simulink model "Robot2_SDT"  (R2025b)
settings: Solver=VariableStepAuto  StartTime=0.0  StopTime=10.0  RelTol=1e-3
values from neighbouring files (symbols this model uses):
  CoM_variation_x = ureal('CoMx',0,"PlusMinus",[-10e-3 10e-3])    [Satellite_Data.m]
  CoM_variation_y = ureal('CoMy',0,"PlusMinus",[-10e-3 10e-3])    [Satellite_Data.m]
  CoM_variation_z = ureal('CoMz',0,"PlusMinus",[-20e-3 20e-3])    [Satellite_Data.m]
  Cross_section_beam = width_beam*height_beam    (= 0.04)    [Satellite_Data.m]
  Iy_beam = (height_beam*width_beam.^3)/12    [Satellite_Data.m]
  Iz_beam = (width_beam*height_beam.^3)/12    [Satellite_Data.m]
  J_B_B = [J_B_Bxx J_B_Bxy J_B_Bxz;         J_B_Bxy J_B_Byy J_B_Byz;         J_B_Bxz J_B_Byz J_B_Bzz]    [Satellite_Data.m]
  J_C_C = [J_C_Cxx J_C_Cxy J_C_Cxz;         J_C_Cxy J_C_Cyy J_C_Cyz;         J_C_Cxz J_C_Cyz J_C_Czz]    [Satellite_Data.m]
  J_P_P = [J_P_Pxx J_P_Pxy J_P_Pxz;         J_P_Pxy J_P_Pyy J_P_Pyz;         J_P_Pxz J_P_Pyz J_P_Pzz]    [Satellite_Data.m]
  length_beam = 4.7    [Satellite_Data.m]
  m_B = ureal('m_B',1000,'percent',10)    [Satellite_Data.m]
  m_C = ureal('m_C',500,'percent',10)    [Satellite_Data.m]
  m_P = ureal('m_P',50,'percent',2)    [Satellite_Data.m]
undefined symbols (not defined in the file or in its folder): InvDyn, InvDynAug, ureal, uss
libraries: RCTblocks x4
settings Model: Creator=l.sekules  LastModifiedBy=l.sekules

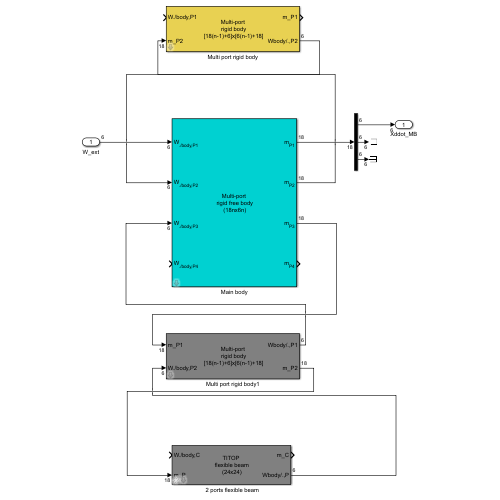
[thumbnail: Simulink's stored preview of the top-level diagram]
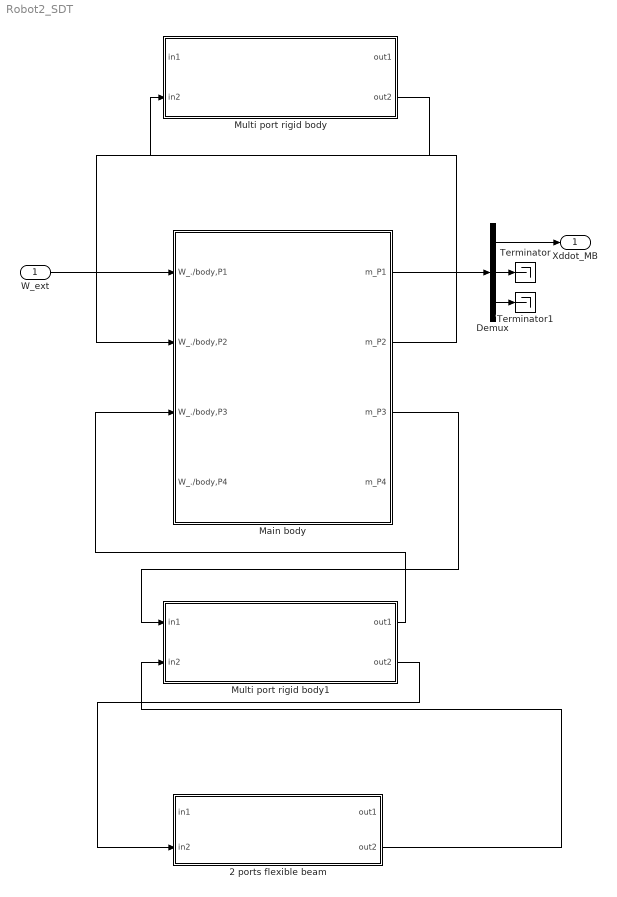
== system Robot2_SDT ==
  W_ext : Inport
  " 2 ports flexible beam" : Subsystem  AncestorBlock=SDTlibV1/6 dof bodies/ 2 ports flexible beam  mask(TITOP Model of a beam){l=length_beam, s=Cross_section_beam, rho=2700, E=7*1e10, Iz=Iz_beam, Iy=Iy_beam, ni=0.33, xi=0.001, free=off, Won=off, uw_var=0, Nflex=10}
      mask prompts: l "lenght along x (m)"; s "cross section  (m^2)"; rho "mass density (Kg/m^3)"; E "Young modulus (N/m^2)"; Iz "second moment of area along z axis, Iz (m^4)"; Iy "second moment of area along y axis Iy, (m^4)"; ni "Poisson coefficient"; xi "damping ratio (nominal clamped-free beam)"; free "Free body at P"; uw_var "uncertainty (d_w, %)"; Nflex "number of flexible mode (Nflex, integer<=10)"
      mask help:
      | 24x24 dynamic model of a uniform beam (along x-axis) between
      |   *  wrench applied to the beam  (input) and motion vector (output) at the "child" (right) tip of the beam
      |   *  motion vector (input)  and wrench applied by the beam at the "parent" (left)  tip of the beam (output).
      | The model is expressed In the beam reference frame (0,x,y,z), see help.
      | Each parameter can be an uncertain parameter declared with "ureal".
      |
      |
      | RK: The last channel associated to parent port P can be inverted to free the body at the point P. In that case, 6 rigid modes (12 integrators) are added in the model to output the motion vector at the point P and the model becomes 36x12.
      mask init:
      | FlexibleBeam2PortAug
      mask Help: web('DocBeam.html','-browser','-browser')
      mask DialogControl Container7 Prompt: Direct uncertainties on flexible mode frequencies
      mask DialogControl Control2 Prompt: Uncertainties on physical parameters (length, mass density, ..) can create huge LFTs.
      mask DialogControl Control3 Prompt: Check this box to overwrite physical parameter uncertainties by a common relative uncertainty (d_w, %) on the first (Nflex) flexible mode frequencies of the clamped at P / free at C beam.
      mask DialogControl Control4 Prompt: The uncertain frequency is named: 'w_name_i' where:
      mask DialogControl Control5 Prompt: * 'name' is the current block name (reduced to its alphanumeric characters).
      mask DialogControl Control6 Prompt: * 'i' is the flexible mode number (increasing frequency order)
      mask Display:
      | if free
      |     disp('TITOP\n flexible beam\n (36x12)')
      | else
      |     disp('TITOP\n flexible beam\n (24x24)')
      | end
      | 
      | port_label('input', 1,'W./body,C')
      | port_label('output',1,'m_C')
      | 
      | if free
      |     port_label('input', 2,'W./body,P')
      |     port_label('output',2,'m_P')
      | else
      |     port_label('input', 2,'m_P')
      |     port_label('output',2,'Wbody/.,P')
      | end
  Demux : Demux  Outputs=3
  Main body : Subsystem  mask(Multi-port rigid body (18nx6n)){m=m_B, Ig=J_B_B, OG=[CoM_variation_x;CoM_variation_y;CoM_variation_z], n=4, OP1=[0;0;0], OP2=[0.35;0;2.5], OP3=[0;0;-2.5], OP4=[1.1;0;0], OP5=[0;0;0]}
      mask prompts: m "Mass (Kg)"; Ig "Inertia (at G, Kg m^2)"; OG "OG (3x1 vector, m)"; n "Number of ports"; OP1 "OP1 (3x1 vector, m)"; OP2 "OP2 (3x1 vector, m)"; OP3 "OP3 (3x1 vector, m)"; OP4 "OP4 (3x1 vector, m)"; OP5 "OP5 (3x1 vector,m)"
      mask help:
      | 18nx6n dynamic model of a rigid body at n given points (ports) between wrenches applied at the n points (input) and the motions vectors at these points (output).
      |
      | 0: the reference point
      | G: the center of mass
      | Pi (i=1:n): the n given connection points (n<6).
      |
      | All parameters are expressed in the body frame.
      | Each parameter can be an uncertain parameter declared with "ureal"
      mask init:
      | MultiPortRigidFreeBody
      mask Help: web('Docmultiportrigidbase.html','-browser','-browser')
      mask TypeOptions n: 1 | 2 | 3 | 4 | 5
      mask DialogControl ParameterGroupVar Prompt: Main parameters
      mask DialogControl port1 Prompt: Port #1
      mask DialogControl port2 Prompt: #2
      mask DialogControl port3 Prompt: #3
      mask DialogControl port4 Prompt: #4
      mask DialogControl port5 Prompt: #5
      mask Display:
      | disp('Multi-port\n rigid free body\n (18nx6n)')
      | for ii=1:n
      |     port_label('input', ii,['W_{./body,P',num2str(ii),'}'],'interpreter','tex')
      |     port_label('output',ii,['m_{P',num2str(ii),'}'],'interpreter','tex')
      | end
  Multi port rigid body : Subsystem  mask(Multi-port rigid body (18(n-1)+6]x[6(n-1)+18])){m=m_C, Ig=J_C_C, OG=[0;0;0], n=2, numinv=2, OP1=[0.75;0;0], OP2=[0;0;(-sqrt(3)-0.5)/2], OP3=[ureal('P3_y',1,'percent',10);0;0], OP4=[0;0;0], OP5=[0;0;0]}
      mask prompts: m "Mass (Kg)"; Ig "Inertia (at G, Kg m^2)"; OG "OG (3x1 vector, m)"; n "Number of ports"; numinv "The single parent port"; OP1 "OP1 (3x1 vector, m)"; OP2 "OP2 (3x1 vector, m)"; OP3 "OP3 (3x1 vector, m)"; OP4 "OP4 (3x1 vector, m)"; OP5 "OP5 (3x1 vector,m)"
      mask help:
      | [18(n-1)+6]x[6(n-1)+18] dynamic model of a rigid body at n given points (ports) between:
      | * the wrenches applied at the n-1 child ports and  the motion vector at a single parent port (inputs).
      | * the motions vectors at the  n-1 child ports and the wrench applied by the rigid body at the parent port (output)
      |
      | 0: the reference point
      | G: the center of mass
      | Pi (i=1:n): the n given connection points (n<6).
      |
      | All parameters are expressed in the body frame.
      | Each parameter can be an uncertain parameter declared with "ureal"
      |
      | The 6x18 channel associated to the single parent port can be any of the ports.
      mask init:
      | MultiPortRigidBodyAug
      mask Help: web('Docmultiportrigidbody.html','-browser','-browser')
      mask TypeOptions n: 1 | 2 | 3 | 4 | 5
      mask TypeOptions numinv: 1 | 2 | 3 | 4 | 5
      mask DialogControl ParameterGroupVar Prompt: Main parameters
      mask DialogControl port1 Prompt: Port #1
      mask DialogControl port2 Prompt: #2
      mask DialogControl port3 Prompt: #3
      mask DialogControl port4 Prompt: #4
      mask DialogControl port5 Prompt: #5
      mask Display:
      | disp('Multi-port\n rigid body\n [18(n-1)+6]x[6(n-1)+18]')
      | if n==1,
      |     if numinv==1,
      |         port_label('input', 1,'m_P')
      |         port_label('output',1,'Wbody/.,P')
      |     else
      |         port_label('input', 1,'W./body,P')
      |         port_label('output',1,'m_P')
      |     end
      | else
      |     for ii=1:n
      |         if numinv==ii,
      |             port_label('output',ii,['Wbody/.,P',num2str(ii)])
      |             port_label('input', ii,['m_P',num2str(ii)])
      |         else
      |             port_label('input', ii,['W./body,P',num2str(ii)])
      |             port_label('output',ii,['m_P',num2str(ii)])
      |         end
      |     end
      | end
  Multi port rigid body1 : Subsystem  mask(Multi-port rigid body (18(n-1)+6]x[6(n-1)+18])){m=m_P, Ig=J_P_P, OG=[0;0;0], n=2, numinv=1, OP1=[0;0;0.2], OP2=[0.1;0;-0.1], OP3=[ureal('P3_y',1,'percent',10);0;0], OP4=[0;0;0], OP5=[0;0;0]}
      mask prompts: m "Mass (Kg)"; Ig "Inertia (at G, Kg m^2)"; OG "OG (3x1 vector, m)"; n "Number of ports"; numinv "The single parent port"; OP1 "OP1 (3x1 vector, m)"; OP2 "OP2 (3x1 vector, m)"; OP3 "OP3 (3x1 vector, m)"; OP4 "OP4 (3x1 vector, m)"; OP5 "OP5 (3x1 vector,m)"
      mask help:
      | [18(n-1)+6]x[6(n-1)+18] dynamic model of a rigid body at n given points (ports) between:
      | * the wrenches applied at the n-1 child ports and  the motion vector at a single parent port (inputs).
      | * the motions vectors at the  n-1 child ports and the wrench applied by the rigid body at the parent port (output)
      |
      | 0: the reference point
      | G: the center of mass
      | Pi (i=1:n): the n given connection points (n<6).
      |
      | All parameters are expressed in the body frame.
      | Each parameter can be an uncertain parameter declared with "ureal"
      |
      | The 6x18 channel associated to the single parent port can be any of the ports.
      mask init:
      | MultiPortRigidBodyAug
      mask Help: web('Docmultiportrigidbody.html','-browser','-browser')
      mask TypeOptions n: 1 | 2 | 3 | 4 | 5
      mask TypeOptions numinv: 1 | 2 | 3 | 4 | 5
      mask DialogControl ParameterGroupVar Prompt: Main parameters
      mask DialogControl port1 Prompt: Port #1
      mask DialogControl port2 Prompt: #2
      mask DialogControl port3 Prompt: #3
      mask DialogControl port4 Prompt: #4
      mask DialogControl port5 Prompt: #5
      mask Display:
      | disp('Multi-port\n rigid body\n [18(n-1)+6]x[6(n-1)+18]')
      | if n==1,
      |     if numinv==1,
      |         port_label('input', 1,'m_P')
      |         port_label('output',1,'Wbody/.,P')
      |     else
      |         port_label('input', 1,'W./body,P')
      |         port_label('output',1,'m_P')
      |     end
      | else
      |     for ii=1:n
      |         if numinv==ii,
      |             port_label('output',ii,['Wbody/.,P',num2str(ii)])
      |             port_label('input', ii,['m_P',num2str(ii)])
      |         else
      |             port_label('input', ii,['W./body,P',num2str(ii)])
      |             port_label('output',ii,['m_P',num2str(ii)])
      |         end
      |     end
      | end
  Terminator : Terminator
  Terminator1 : Terminator
  Xddot_MB : Outport
  wires:
  W_ext/1 -> Main body/1(W_./body,P1)
  Main body/2(m_P2) -> Multi port rigid body/2(in2)
  Multi port rigid body/2(out2) -> Main body/2(W_./body,P2)
  Main body/3(m_P3) -> Multi port rigid body1/1(in1)
  Multi port rigid body1/1(out1) -> Main body/3(W_./body,P3)
  Main body/1(m_P1) -> Demux/1
  Demux/1 -> Xddot_MB/1
  Demux/2 -> Terminator/1
  Demux/3 -> Terminator1/1
  Multi port rigid body1/2(out2) -> " 2 ports flexible beam"/2(in2)
  " 2 ports flexible beam"/2(out2) -> Multi port rigid body1/2(in2)

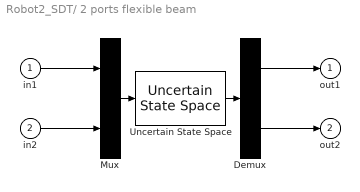
== system Robot2_SDT/ 2 ports flexible beam ==
  in1 : Inport  PortDimensions=6
  in2 : Inport  Port=2  PortDimensions=18
  Demux : Demux  Outputs=[18 6]
      settings: DisplayOption=none
  Mux : Mux  Inputs=[6 18]
  Uncertain State Space : RCTblocks/Uncertain State Space  Tag=USS  USystem=TITOPBEAM  UValue=[]  X0=[]  uX0=[]
  out1 : Outport  VectorParamsAs1DForOutWhenUnconnected=off
  out2 : Outport  Port=2  VectorParamsAs1DForOutWhenUnconnected=off
  wires:
  Mux/1 -> Uncertain State Space/1
  Uncertain State Space/1 -> Demux/1
  in1/1 -> Mux/1
  Demux/1 -> out1/1
  in2/1 -> Mux/2
  Demux/2 -> out2/1

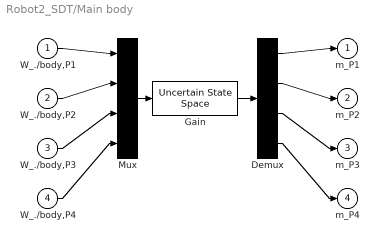
== system Robot2_SDT/Main body ==
  W_./body,P1 : Inport  PortDimensions=6
  W_./body,P2 : Inport  Port=2  PortDimensions=6
  W_./body,P3 : Inport  Port=3  PortDimensions=6
  W_./body,P4 : Inport  Port=4  PortDimensions=6
  Demux : Demux  Outputs=[18 18 18 18]
  Gain : RCTblocks/Uncertain State Space  Tag=USS  USystem=uss(InvDyn)  UValue=[]  X0=[]  uX0=[]
  Mux : Mux  Inputs=[6 6 6 6]
  m_P1 : Outport
  m_P2 : Outport  Port=2
  m_P3 : Outport  Port=3
  m_P4 : Outport  Port=4
  wires:
  Mux/1 -> Gain/1
  Gain/1 -> Demux/1
  W_./body,P1/1 -> Mux/1
  Demux/1 -> m_P1/1
  W_./body,P2/1 -> Mux/2
  Demux/2 -> m_P2/1
  W_./body,P3/1 -> Mux/3
  Demux/3 -> m_P3/1
  W_./body,P4/1 -> Mux/4
  Demux/4 -> m_P4/1

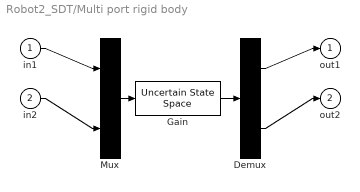
== system Robot2_SDT/Multi port rigid body ==
  in1 : Inport  PortDimensions=6
  in2 : Inport  Port=2  PortDimensions=18
  Demux : Demux  Outputs=[ 18 6]
  Gain : RCTblocks/Uncertain State Space  Tag=USS  USystem=uss(InvDynAug)  UValue=[]  X0=[]  uX0=[]
  Mux : Mux  Inputs=[ 6 18]
  out1 : Outport
  out2 : Outport  Port=2
  wires:
  Mux/1 -> Gain/1
  Gain/1 -> Demux/1
  in1/1 -> Mux/1
  Demux/1 -> out1/1
  in2/1 -> Mux/2
  Demux/2 -> out2/1

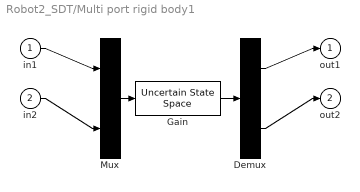
== system Robot2_SDT/Multi port rigid body1 ==
  in1 : Inport  PortDimensions=18
  in2 : Inport  Port=2  PortDimensions=6
  Demux : Demux  Outputs=[ 6 18]
  Gain : RCTblocks/Uncertain State Space  Tag=USS  USystem=uss(InvDynAug)  UValue=[]  X0=[]  uX0=[]
  Mux : Mux  Inputs=[ 18 6]
  out1 : Outport
  out2 : Outport  Port=2
  wires:
  Demux/2 -> out2/1
  in2/1 -> Mux/2
  Demux/1 -> out1/1
  in1/1 -> Mux/1
  Gain/1 -> Demux/1
  Mux/1 -> Gain/1
